simulink model "sistemas_segundo_orden"  (Simulink 7.7)
settings: Solver=ode3  StartTime=0.0  StopTime=20.0  FixedStep=0.01  MaxStep=0.01  MinStep=0.01  RelTol=0.001  AbsTol=0.001
settings Model: Creator=juen  LastModifiedBy=juen
settings SolverCC: InitialStep=0.01
settings DataIOCC: LimitDataPoints=off

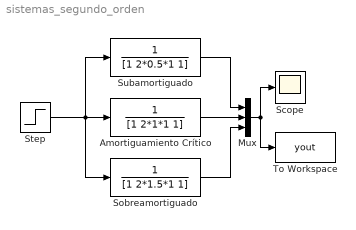
== system sistemas_segundo_orden ==
  Amortiguamiento Crítico : TransferFcn  Denominator=[1 2*1*1 1]
  Mux : Mux  Inputs=3
  Scope : Scope
  Sobreamortiguado : TransferFcn  Denominator=[1 2*1.5*1 1]
  Step : Step  SampleTime=0
  Subamortiguado : TransferFcn  Denominator=[1 2*0.5*1 1]
  To Workspace : ToWorkspace  VariableName=yout  SampleTime=-1  SaveFormat=Structure With Time
  wires:
  Step/1 -> Subamortiguado/1, Amortiguamiento Crítico/1, Sobreamortiguado/1
  Amortiguamiento Crítico/1 -> Mux/2
  Subamortiguado/1 -> Mux/1
  Sobreamortiguado/1 -> Mux/3
  Mux/1 -> To Workspace/1, Scope/1
